simulink model "ACAC"  (R2022b)
settings: Solver=VariableStepAuto  StartTime=0.0  StopTime=0.5  RelTol=1e-3
libraries: spsVoltageMeasurementLib x2, dspsigops x2, spsThyristorLib x2, spsACVoltageSourceLib x1, spsCurrentMeasurementLib x1, simulink x1, spsSeriesRLCBranchLib x1, spspowerguiLib x1
settings Model: Creator=rames  LastModifiedBy=rishi kumar singh

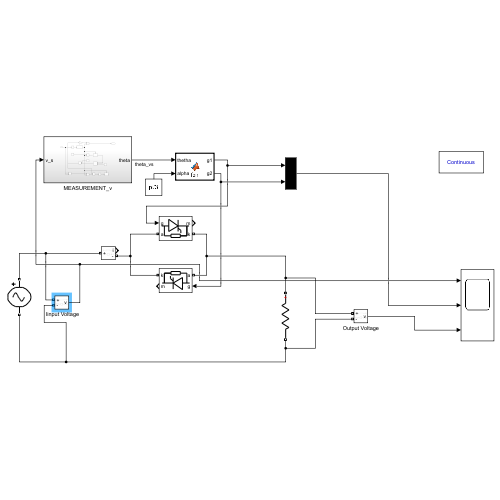
[thumbnail: Simulink's stored preview of the top-level diagram]
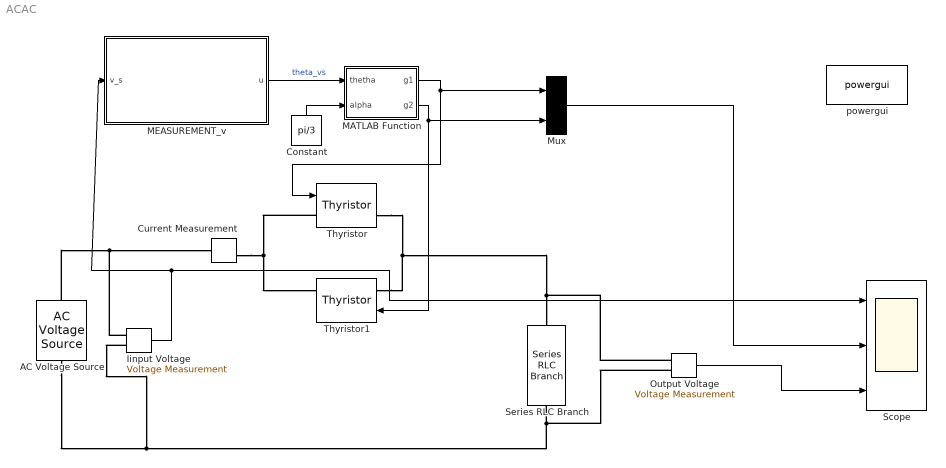
== system ACAC ==
  " Iinput Voltage" : spsVoltageMeasurementLib/Voltage Measurement  PhasorSimulation=off  OutputType=Complex  PSBequivalent=0
  AC Voltage Source : spsACVoltageSourceLib/AC Voltage Source  Amplitude=230*sqrt(2)  Phase=0  Frequency=50  SampleTime=0  Measurements=None  BusType=swing  Pref=10e3  Qref=0  Qmin=-inf  Qmax=+inf
  Constant : Constant  Value=pi/3
  Current Measurement : spsCurrentMeasurementLib/Current Measurement  PhasorSimulation=off  OutputType=Complex  PSBequivalent=0
  MATLAB Function : MATLAB Function  TreatAsAtomicUnit=on
  MEASUREMENT_v : Subsystem
  Mux : Mux  Inputs=2
  Output Voltage : spsVoltageMeasurementLib/Voltage Measurement  PhasorSimulation=off  OutputType=Complex  PSBequivalent=0
  Scope : Scope  NumInputPorts=3
  Series RLC Branch : spsSeriesRLCBranchLib/Series RLC Branch  LConnTagsString=__new0  RConnTagsString=__new0  BranchType=R  Resistance=10  Inductance=1e-3  SetiL0=off  InitialCurrent=0  Capacitance=1e-6  Setx0=off  InitialVoltage=0  Measurements=None
  Thyristor : spsThyristorLib/Thyristor  Ron=0.001  Lon=0  Vf=0.8  IC=0  Rs=500  Cs=250e-9  Measurements=on
  Thyristor1 : spsThyristorLib/Thyristor  Ron=0.001  Lon=0  Vf=0.8  IC=0  Rs=500  Cs=250e-9  Measurements=on
  powergui : spspowerguiLib/powergui  Priority=1  SimulationMode=Continuous  SampleTime=50e-6  frequency=60  Iterations=50  frequencyindice=50  Pbase=100e6  ErrMax=1e-4  UnitsV=kV  UnitsW=MW  buscounter=0  FunctionMessages=off  echomessages=off  EnableUseOfTLC=off  CurrentSourceSwitches=off  DisableSnubberDevices=off  DisableRonSwitches=off  DisableVfSwitches=off  DisplayEquations=off  AutomaticDiscreteSolvers=off  SolverType=Tustin/Backward Euler (TBE)  Interpol=off  ExternalGateDelay=off  methode=off  Ts=100  x0status=blocks  SPID=on  SwTol=0  HookPort=off  NonlinearTolerance=1e-4  nMaxIteration=100  ContinueOnMaxIteration=off  RestoreLinks=warning  ResistiveCurrentMeasurement=off  Frange=[0:2:500]  Ylog=off  Xlog=on  ShowGrid=off  save=off  variable=ZData  structure=0  ZoomFFT=off  StartTime=0.0  cycles=1  DisplayStyle=1  fundamental=60  FreqAxis=off  MaxFrequency=1000  frequencyindicesteady=1  RmsSteady=1  display=off
  wires:
  " Iinput Voltage"/1 -> MEASUREMENT_v/1(v_s), Scope/1
  MEASUREMENT_v/1(u) -> MATLAB Function/1(thetha)  "theta_vs"
  Constant/1 -> MATLAB Function/2(alpha)
  MATLAB Function/1(g1) -> Mux/1, Thyristor/1
  MATLAB Function/2(g2) -> Mux/2, Thyristor1/1
  Mux/1 -> Scope/2
  Output Voltage/1 -> Scope/3
  connections:
  " Iinput Voltage"/LConn2 -- Output Voltage/LConn2 -- Series RLC Branch/RConn1 -- AC Voltage Source/LConn1
  " Iinput Voltage"/LConn1 -- Current Measurement/LConn1 -- AC Voltage Source/RConn1
  Output Voltage/LConn1 -- Thyristor/RConn1 -- Thyristor1/LConn1 -- Series RLC Branch/LConn1
  Current Measurement/RConn1 -- Thyristor/LConn1 -- Thyristor1/RConn1

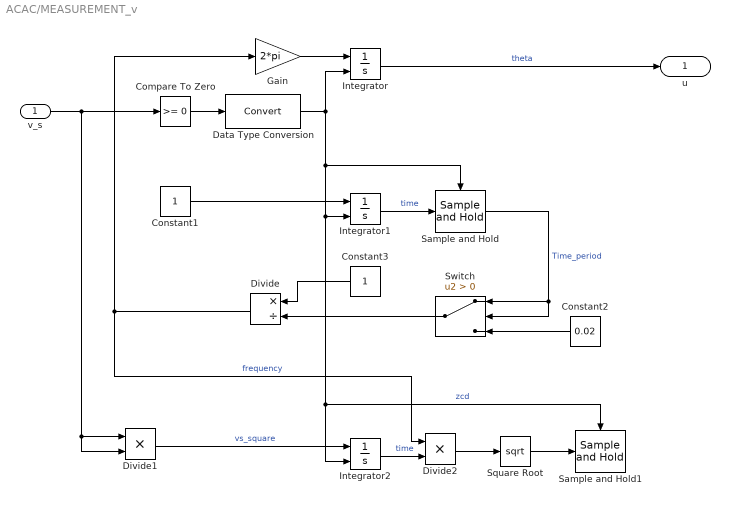
== system ACAC/MEASUREMENT_v ==
  v_s : Inport
  Compare To Zero : simulink/Logic and Bit Operations/Compare To Zero  relop=>=  OutDataTypeStr=boolean
  Constant1 : Constant
  Constant2 : Constant  Value=0.02
  Constant3 : Constant
  Data Type Conversion : DataTypeConversion  SaturateOnIntegerOverflow=off  RndMeth=Floor
  Divide : Product  Inputs=*/
  Divide1 : Product  Inputs=**
  Divide2 : Product  Inputs=**
  Gain : Gain  Gain=2*pi
  Integrator : Integrator  ExternalReset=rising
  Integrator1 : Integrator  ExternalReset=rising
  Integrator2 : Integrator  ExternalReset=rising
  Sample and Hold : dspsigops/Sample and Hold  trig=Rising edge  initCond=0  latchinput=on
  Sample and Hold1 : dspsigops/Sample and Hold  trig=Rising edge  initCond=0  latchinput=on
  Square Root : Sqrt
  Switch : Switch  Criteria=u2 > Threshold  SaturateOnIntegerOverflow=off  InputSameDT=off
  u : Outport
  wires:
  Compare To Zero/1 -> Data Type Conversion/1
  Constant3/1 -> Divide/1
  Integrator/1 -> u/1  "theta"
  Divide/1 -> Gain/1, Divide2/1  "frequency"
  Data Type Conversion/1 -> Integrator1/2, Sample and Hold1/Trigger, Integrator2/2, Sample and Hold/Trigger, Integrator/2  "zcd"
  Gain/1 -> Integrator/1
  Sample and Hold/1 -> Switch/2, Switch/1  "Time_period"
  Constant2/1 -> Switch/3
  Constant1/1 -> Integrator1/1
  Integrator1/1 -> Sample and Hold/1  "time"
  Switch/1 -> Divide/2
  v_s/1 -> Divide1/2, Divide1/1, Compare To Zero/1
  Divide1/1 -> Integrator2/1  "vs_square"
  Integrator2/1 -> Divide2/2  "time"
  Divide2/1 -> Square Root/1
  Square Root/1 -> Sample and Hold1/1

== matlab function ACAC/MATLAB Function ==
  data: thetha input; alpha input; g1 output; g2 output
function [g1,g2] = fcn(thetha,alpha)
g1=0;
g2=0;
if(thetha>=0 && thetha<alpha)
    g1=0;
    g2=0;
end
if(thetha>=alpha && thetha<pi)
    g1=1;
    g2=0;
end
if(thetha>=pi && thetha<(pi+alpha))
    g1=0;
    g2=0;
end
if(thetha>=(pi+alpha) && thetha<2*pi)
    g1=0;
    g2=1;
end
